simulink model "verify_tau"  (R2025b)
settings: Solver=ode4  StartTime=0.0  StopTime=8.5  FixedStep=0.01  RelTol=1e-5  AbsTol=1e-6
libraries: sldvlib x1
settings Model: Creator=Deermste  LastModifiedBy=Deermste
settings ConfigComp: DVMode=PropertyProving  DVMaxProcessTime=300.0  DVMaxTestCaseSteps=10000.0  DVTestSuiteOptimization=Auto  DVAbsoluteTolerance=1.0e-5  DVDefectChecker=on  DVDetectOutOfBounds=on  DVMaxViolationSteps=20.0  DVModelReferenceHarness=on  DVHarnessSource=Signal Editor  DVActiveTab=0.0

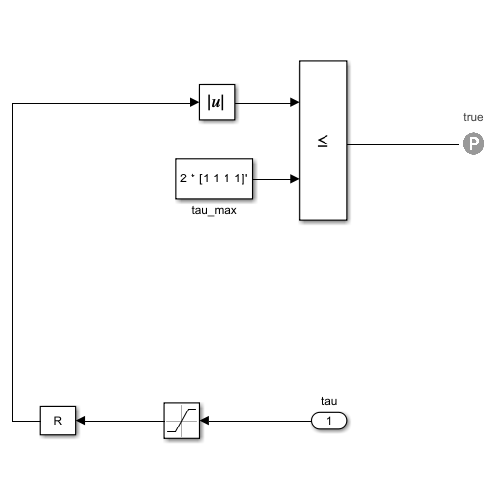
[thumbnail: Simulink's stored preview of the top-level diagram]
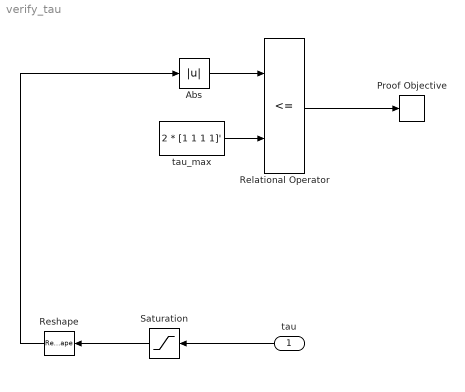
== system verify_tau ==
  tau : Inport
  Abs : Abs  SaturateOnIntegerOverflow=off
  Proof Objective : sldvlib/Objectives and Constraints/Proof Objective  enabled=on  customAVTBlockType=Proof Objective  intervals=true  dispValues=on  outEnabled=off  enableStopSim=off
      settings: AttributesFormatString=%<intervals>
  Relational Operator : RelationalOperator  Operator=<=  OutDataTypeStr=boolean  RndMeth=Simplest  InputSameDT=off
  Reshape : Reshape  OutputDimensionality=Customize  OutputDimensions=[4, 1]
  Saturation : Saturate  UpperLimit=2  LowerLimit=-2
  tau_max : Constant  Value=2 * [1 1 1 1]'
  wires:
  Reshape/1 -> Abs/1
  Saturation/1 -> Reshape/1
  tau/1 -> Saturation/1
  Abs/1 -> Relational Operator/1
  tau_max/1 -> Relational Operator/2
  Relational Operator/1 -> Proof Objective/1
